simulink model "TST_CrCUI"  (R2016b)
settings: Solver=FixedStepDiscrete  StartTime=0.0  StopTime=simTime  FixedStep=sampleTime  RelTol=1e-3
values from neighbouring files (symbols this model uses):
  testCase = 1    [initTST_CrCUI_001.m]
libraries: simulink x4, UnitTest_Lib x1
settings Model: Creator=guanxiaoxing  LastModifiedBy=guanxiaoxing
settings DebuggingCC: SignalRangeChecking=error

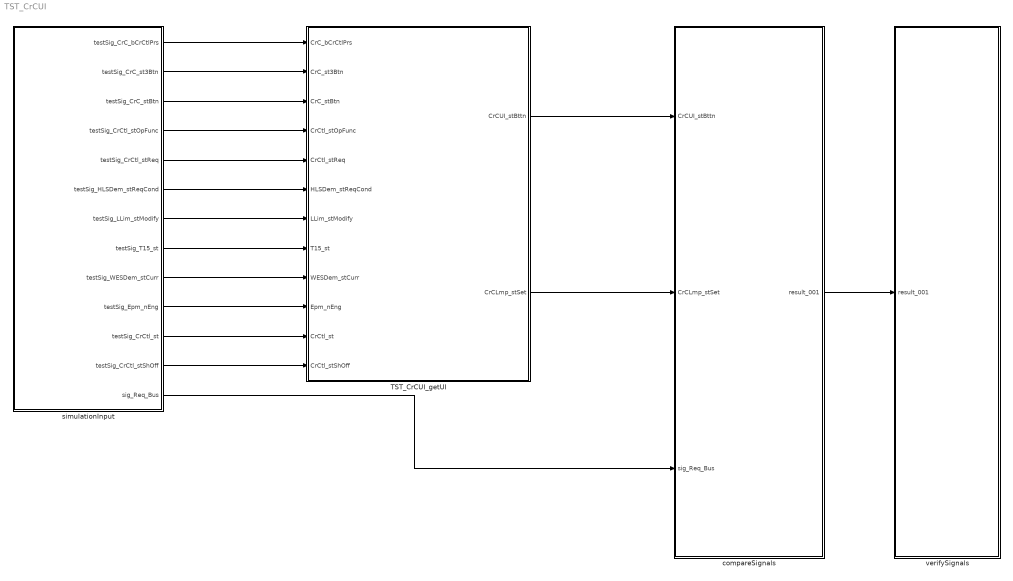
== system TST_CrCUI ==
  TST_CrCUI_getUI : Subsystem
  compareSignals : Subsystem
  simulationInput : Subsystem
  verifySignals : Subsystem
  wires:
  simulationInput/1(testSig_CrC_bCrCtlPrs) -> TST_CrCUI_getUI/1(CrC_bCrCtlPrs)
  simulationInput/2(testSig_CrC_st3Btn) -> TST_CrCUI_getUI/2(CrC_st3Btn)
  simulationInput/3(testSig_CrC_stBtn) -> TST_CrCUI_getUI/3(CrC_stBtn)
  simulationInput/4(testSig_CrCtl_stOpFunc) -> TST_CrCUI_getUI/4(CrCtl_stOpFunc)
  simulationInput/5(testSig_CrCtl_stReq) -> TST_CrCUI_getUI/5(CrCtl_stReq)
  simulationInput/6(testSig_HLSDem_stReqCond) -> TST_CrCUI_getUI/6(HLSDem_stReqCond)
  simulationInput/7(testSig_LLim_stModify) -> TST_CrCUI_getUI/7(LLim_stModify)
  simulationInput/8(testSig_T15_st) -> TST_CrCUI_getUI/8(T15_st)
  simulationInput/9(testSig_WESDem_stCurr) -> TST_CrCUI_getUI/9(WESDem_stCurr)
  simulationInput/10(testSig_Epm_nEng) -> TST_CrCUI_getUI/10(Epm_nEng)
  simulationInput/11(testSig_CrCtl_st) -> TST_CrCUI_getUI/11(CrCtl_st)
  simulationInput/12(testSig_CrCtl_stShOff) -> TST_CrCUI_getUI/12(CrCtl_stShOff)
  TST_CrCUI_getUI/1(CrCUI_stBttn) -> compareSignals/1(CrCUI_stBttn)
  TST_CrCUI_getUI/2(CrCLmp_stSet) -> compareSignals/2(CrCLmp_stSet)
  simulationInput/13(sig_Req_Bus) -> compareSignals/3(sig_Req_Bus)
  compareSignals/1(result_001) -> verifySignals/1(result_001)

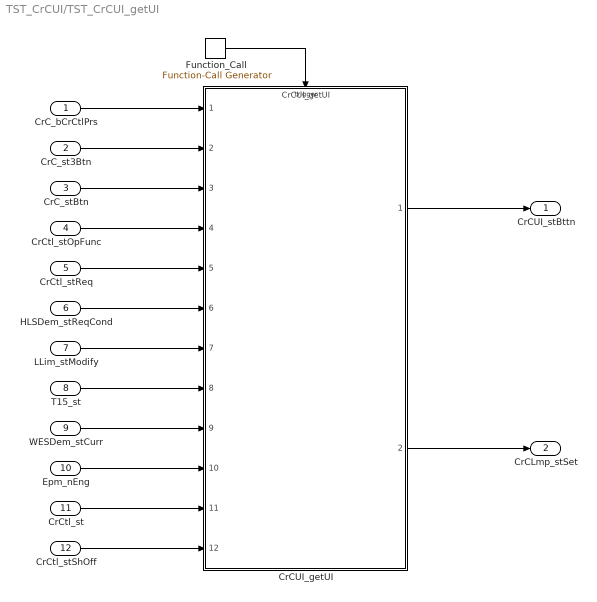
== system TST_CrCUI/TST_CrCUI_getUI ==
  CrC_bCrCtlPrs : Inport
  CrC_st3Btn : Inport  Port=2
  CrC_stBtn : Inport  Port=3
  CrCtl_stOpFunc : Inport  Port=4
  CrCtl_stReq : Inport  Port=5
  HLSDem_stReqCond : Inport  Port=6
  LLim_stModify : Inport  Port=7
  T15_st : Inport  Port=8
  WESDem_stCurr : Inport  Port=9
  Epm_nEng : Inport  Port=10
  CrCtl_st : Inport  Port=11
  CrCtl_stShOff : Inport  Port=12
  CrCUI_getUI : ModelReference  ModelNameDialog=CrCUI_getUI  SimulationMode=Normal  ModelReferenceVersion=1.56  TriggerPortName=function  TriggerPortTriggerType=function-call  TriggerPortStatesWhenEnabling=held
  Function_Call : simulink/Ports & Subsystems/Function-Call Generator  sample_time=sampleTime  numberOfIterations=1
  CrCUI_stBttn : Outport
  CrCLmp_stSet : Outport  Port=2
  wires:
  Function_Call/1 -> CrCUI_getUI/Trigger
  CrC_bCrCtlPrs/1 -> CrCUI_getUI/1
  CrC_st3Btn/1 -> CrCUI_getUI/2
  CrC_stBtn/1 -> CrCUI_getUI/3
  CrCtl_stOpFunc/1 -> CrCUI_getUI/4
  CrCtl_stReq/1 -> CrCUI_getUI/5
  HLSDem_stReqCond/1 -> CrCUI_getUI/6
  LLim_stModify/1 -> CrCUI_getUI/7
  T15_st/1 -> CrCUI_getUI/8
  WESDem_stCurr/1 -> CrCUI_getUI/9
  Epm_nEng/1 -> CrCUI_getUI/10
  CrCtl_st/1 -> CrCUI_getUI/11
  CrCtl_stShOff/1 -> CrCUI_getUI/12
  CrCUI_getUI/1 -> CrCUI_stBttn/1
  CrCUI_getUI/2 -> CrCLmp_stSet/1

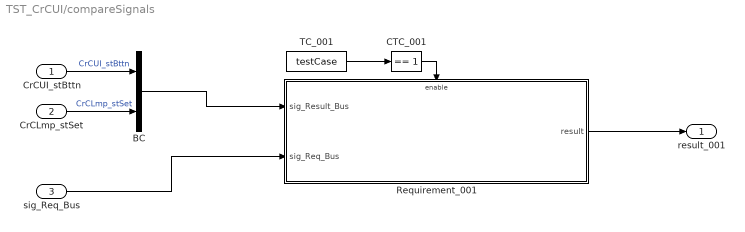
== system TST_CrCUI/compareSignals ==
  CrCUI_stBttn : Inport
  CrCLmp_stSet : Inport  Port=2
  sig_Req_Bus : Inport  Port=3
  BC : BusCreator  Inputs=2
  CTC_001 : simulink/Logic and Bit Operations/Compare To Constant  relop===  const=1  OutDataTypeStr=boolean
  Requirement_001 : Subsystem
  TC_001 : Constant  Value=testCase
  result_001 : Outport
  wires:
  CrCUI_stBttn/1 -> BC/1  "CrCUI_stBttn"
  CrCLmp_stSet/1 -> BC/2  "CrCLmp_stSet"
  TC_001/1 -> CTC_001/1
  CTC_001/1 -> Requirement_001/Enable
  sig_Req_Bus/1 -> Requirement_001/2(sig_Req_Bus)
  BC/1 -> Requirement_001/1(sig_Result_Bus)
  Requirement_001/1(result) -> result_001/1

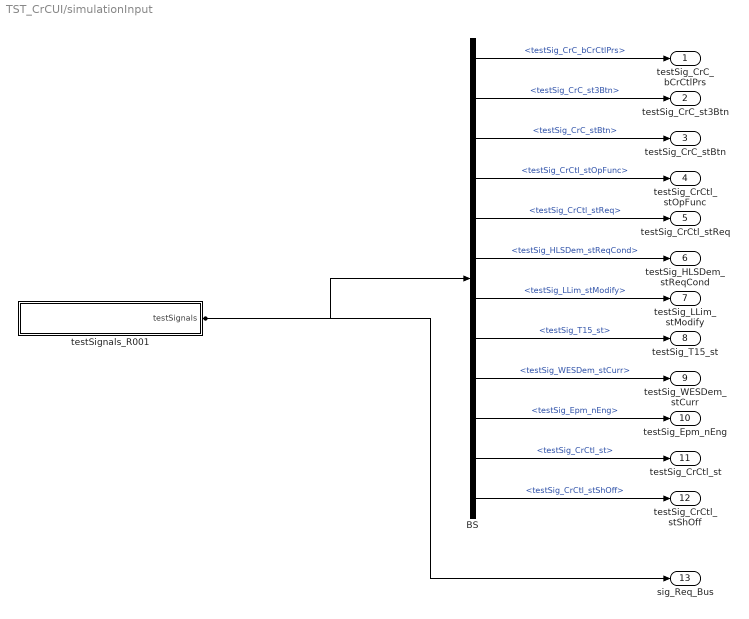
== system TST_CrCUI/simulationInput ==
  BS : BusSelector  OutputSignals=testSig_CrC_bCrCtlPrs,testSig_CrC_st3Btn,testSig_CrC_stBtn,testSig_CrCtl_stOpFunc,testSig_CrCtl_stReq,testSig_HLSDem_stReqCond,testSig_LLim_stModify,testSig_T15_st,testSig_WESDem_stCurr,testSig_Epm_nEng,testSig_CrCtl_st,testSig_CrCtl_stShOff
  testSignals_R001 : Subsystem
  testSig_CrC_bCrCtlPrs : Outport
  testSig_CrC_st3Btn : Outport  Port=2
  testSig_CrC_stBtn : Outport  Port=3
  testSig_CrCtl_stOpFunc : Outport  Port=4
  testSig_CrCtl_stReq : Outport  Port=5
  testSig_HLSDem_stReqCond : Outport  Port=6
  testSig_LLim_stModify : Outport  Port=7
  testSig_T15_st : Outport  Port=8
  testSig_WESDem_stCurr : Outport  Port=9
  testSig_Epm_nEng : Outport  Port=10
  testSig_CrCtl_st : Outport  Port=11
  testSig_CrCtl_stShOff : Outport  Port=12
  sig_Req_Bus : Outport  Port=13
  wires:
  BS/1 -> testSig_CrC_bCrCtlPrs/1  "<testSig_CrC_bCrCtlPrs>"
  BS/2 -> testSig_CrC_st3Btn/1  "<testSig_CrC_st3Btn>"
  BS/3 -> testSig_CrC_stBtn/1  "<testSig_CrC_stBtn>"
  BS/4 -> testSig_CrCtl_stOpFunc/1  "<testSig_CrCtl_stOpFunc>"
  BS/5 -> testSig_CrCtl_stReq/1  "<testSig_CrCtl_stReq>"
  BS/6 -> testSig_HLSDem_stReqCond/1  "<testSig_HLSDem_stReqCond>"
  BS/7 -> testSig_LLim_stModify/1  "<testSig_LLim_stModify>"
  BS/8 -> testSig_T15_st/1  "<testSig_T15_st>"
  BS/9 -> testSig_WESDem_stCurr/1  "<testSig_WESDem_stCurr>"
  BS/10 -> testSig_Epm_nEng/1  "<testSig_Epm_nEng>"
  BS/11 -> testSig_CrCtl_st/1  "<testSig_CrCtl_st>"
  BS/12 -> testSig_CrCtl_stShOff/1  "<testSig_CrCtl_stShOff>"
  testSignals_R001/1(testSignals) -> BS/1, sig_Req_Bus/1

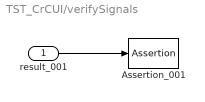
== system TST_CrCUI/verifySignals ==
  result_001 : Inport
  Assertion_001 : Assertion  Enabled=off
  wires:
  result_001/1 -> Assertion_001/1

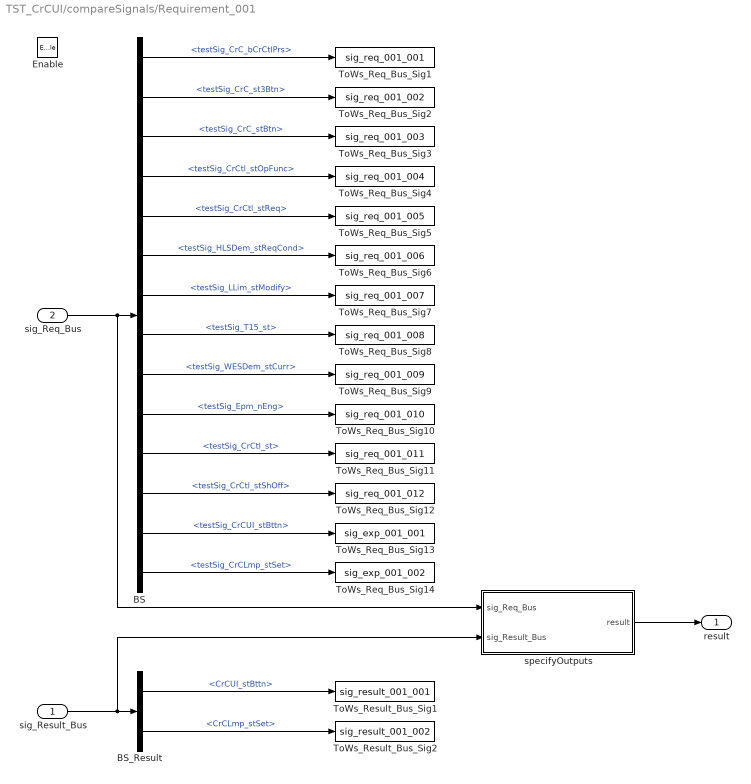
== system TST_CrCUI/compareSignals/Requirement_001 ==
  sig_Result_Bus : Inport
  sig_Req_Bus : Inport  Port=2
  Enable : EnablePort
  BS : BusSelector  OutputSignals=testSig_CrC_bCrCtlPrs,testSig_CrC_st3Btn,testSig_CrC_stBtn,testSig_CrCtl_stOpFunc,testSig_CrCtl_stReq,testSig_HLSDem_stReqCond,testSig_LLim_stModify,testSig_T15_st,testSig_WESDem_stCurr,testSig_Epm_nEng,testSig_CrCtl_st,testSig_CrCtl_stShOff,testSig_CrCUI_stBttn,testSig_CrCLmp_stSet
  BS_Result : BusSelector  OutputSignals=CrCUI_stBttn,CrCLmp_stSet
  ToWs_Req_Bus_Sig1 : ToWorkspace  VariableName=sig_req_001_001  SaveFormat=Structure With Time
  ToWs_Req_Bus_Sig10 : ToWorkspace  VariableName=sig_req_001_010  SaveFormat=Structure With Time
  ToWs_Req_Bus_Sig11 : ToWorkspace  VariableName=sig_req_001_011  SaveFormat=Structure With Time
  ToWs_Req_Bus_Sig12 : ToWorkspace  VariableName=sig_req_001_012  SaveFormat=Structure With Time
  ToWs_Req_Bus_Sig13 : ToWorkspace  VariableName=sig_exp_001_001  SaveFormat=Structure With Time
  ToWs_Req_Bus_Sig14 : ToWorkspace  VariableName=sig_exp_001_002  SaveFormat=Structure With Time
  ToWs_Req_Bus_Sig2 : ToWorkspace  VariableName=sig_req_001_002  SaveFormat=Structure With Time
  ToWs_Req_Bus_Sig3 : ToWorkspace  VariableName=sig_req_001_003  SaveFormat=Structure With Time
  ToWs_Req_Bus_Sig4 : ToWorkspace  VariableName=sig_req_001_004  SaveFormat=Structure With Time
  ToWs_Req_Bus_Sig5 : ToWorkspace  VariableName=sig_req_001_005  SaveFormat=Structure With Time
  ToWs_Req_Bus_Sig6 : ToWorkspace  VariableName=sig_req_001_006  SaveFormat=Structure With Time
  ToWs_Req_Bus_Sig7 : ToWorkspace  VariableName=sig_req_001_007  SaveFormat=Structure With Time
  ToWs_Req_Bus_Sig8 : ToWorkspace  VariableName=sig_req_001_008  SaveFormat=Structure With Time
  ToWs_Req_Bus_Sig9 : ToWorkspace  VariableName=sig_req_001_009  SaveFormat=Structure With Time
  ToWs_Result_Bus_Sig1 : ToWorkspace  VariableName=sig_result_001_001  SaveFormat=Structure With Time
  ToWs_Result_Bus_Sig2 : ToWorkspace  VariableName=sig_result_001_002  SaveFormat=Structure With Time
  specifyOutputs : Subsystem
  result : Outport
  wires:
  sig_Req_Bus/1 -> BS/1, specifyOutputs/1(sig_Req_Bus)
  BS/1 -> ToWs_Req_Bus_Sig1/1  "<testSig_CrC_bCrCtlPrs>"
  BS/2 -> ToWs_Req_Bus_Sig2/1  "<testSig_CrC_st3Btn>"
  BS/3 -> ToWs_Req_Bus_Sig3/1  "<testSig_CrC_stBtn>"
  BS/4 -> ToWs_Req_Bus_Sig4/1  "<testSig_CrCtl_stOpFunc>"
  BS/5 -> ToWs_Req_Bus_Sig5/1  "<testSig_CrCtl_stReq>"
  BS/6 -> ToWs_Req_Bus_Sig6/1  "<testSig_HLSDem_stReqCond>"
  BS/7 -> ToWs_Req_Bus_Sig7/1  "<testSig_LLim_stModify>"
  BS/8 -> ToWs_Req_Bus_Sig8/1  "<testSig_T15_st>"
  BS/9 -> ToWs_Req_Bus_Sig9/1  "<testSig_WESDem_stCurr>"
  BS/10 -> ToWs_Req_Bus_Sig10/1  "<testSig_Epm_nEng>"
  BS/11 -> ToWs_Req_Bus_Sig11/1  "<testSig_CrCtl_st>"
  BS/12 -> ToWs_Req_Bus_Sig12/1  "<testSig_CrCtl_stShOff>"
  BS/13 -> ToWs_Req_Bus_Sig13/1  "<testSig_CrCUI_stBttn>"
  BS/14 -> ToWs_Req_Bus_Sig14/1  "<testSig_CrCLmp_stSet>"
  sig_Result_Bus/1 -> BS_Result/1, specifyOutputs/2(sig_Result_Bus)
  BS_Result/1 -> ToWs_Result_Bus_Sig1/1  "<CrCUI_stBttn>"
  BS_Result/2 -> ToWs_Result_Bus_Sig2/1  "<CrCLmp_stSet>"
  specifyOutputs/1(result) -> result/1

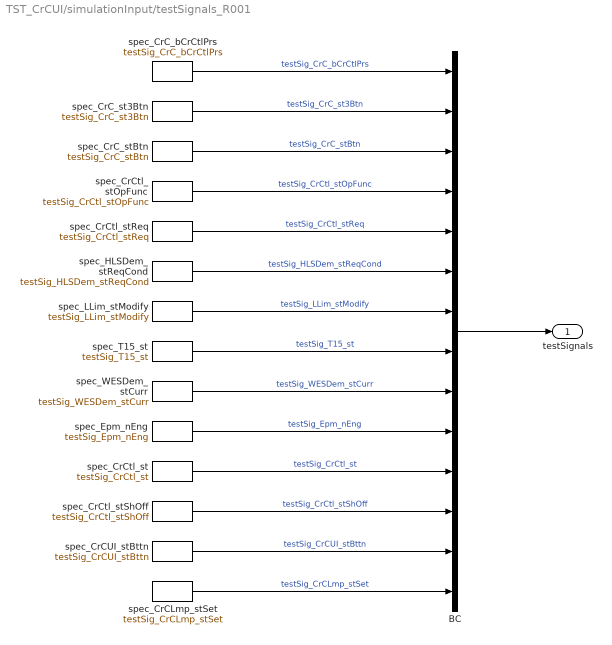
== system TST_CrCUI/simulationInput/testSignals_R001 ==
  BC : BusCreator  Inputs=14
  spec_CrCLmp_stSet : FromWorkspace  VariableName=testSig_CrCLmp_stSet  Interpolate=off  OutputAfterFinalValue=Holding final value
  spec_CrCUI_stBttn : FromWorkspace  VariableName=testSig_CrCUI_stBttn  Interpolate=off  OutputAfterFinalValue=Holding final value
  spec_CrC_bCrCtlPrs : FromWorkspace  VariableName=testSig_CrC_bCrCtlPrs  Interpolate=off  OutputAfterFinalValue=Holding final value
  spec_CrC_st3Btn : FromWorkspace  VariableName=testSig_CrC_st3Btn  Interpolate=off  OutputAfterFinalValue=Holding final value
  spec_CrC_stBtn : FromWorkspace  VariableName=testSig_CrC_stBtn  Interpolate=off  OutputAfterFinalValue=Holding final value
  spec_CrCtl_st : FromWorkspace  VariableName=testSig_CrCtl_st  Interpolate=off  OutputAfterFinalValue=Holding final value
  spec_CrCtl_stOpFunc : FromWorkspace  VariableName=testSig_CrCtl_stOpFunc  Interpolate=off  OutputAfterFinalValue=Holding final value
  spec_CrCtl_stReq : FromWorkspace  VariableName=testSig_CrCtl_stReq  Interpolate=off  OutputAfterFinalValue=Holding final value
  spec_CrCtl_stShOff : FromWorkspace  VariableName=testSig_CrCtl_stShOff  Interpolate=off  OutputAfterFinalValue=Holding final value
  spec_Epm_nEng : FromWorkspace  VariableName=testSig_Epm_nEng  Interpolate=off  OutputAfterFinalValue=Holding final value
  spec_HLSDem_stReqCond : FromWorkspace  VariableName=testSig_HLSDem_stReqCond  Interpolate=off  OutputAfterFinalValue=Holding final value
  spec_LLim_stModify : FromWorkspace  VariableName=testSig_LLim_stModify  Interpolate=off  OutputAfterFinalValue=Holding final value
  spec_T15_st : FromWorkspace  VariableName=testSig_T15_st  Interpolate=off  OutputAfterFinalValue=Holding final value
  spec_WESDem_stCurr : FromWorkspace  VariableName=testSig_WESDem_stCurr  Interpolate=off  OutputAfterFinalValue=Holding final value
  testSignals : Outport
  wires:
  BC/1 -> testSignals/1
  spec_CrC_bCrCtlPrs/1 -> BC/1  "testSig_CrC_bCrCtlPrs"
  spec_CrC_st3Btn/1 -> BC/2  "testSig_CrC_st3Btn"
  spec_CrC_stBtn/1 -> BC/3  "testSig_CrC_stBtn"
  spec_CrCtl_stOpFunc/1 -> BC/4  "testSig_CrCtl_stOpFunc"
  spec_CrCtl_stReq/1 -> BC/5  "testSig_CrCtl_stReq"
  spec_HLSDem_stReqCond/1 -> BC/6  "testSig_HLSDem_stReqCond"
  spec_LLim_stModify/1 -> BC/7  "testSig_LLim_stModify"
  spec_T15_st/1 -> BC/8  "testSig_T15_st"
  spec_WESDem_stCurr/1 -> BC/9  "testSig_WESDem_stCurr"
  spec_Epm_nEng/1 -> BC/10  "testSig_Epm_nEng"
  spec_CrCtl_st/1 -> BC/11  "testSig_CrCtl_st"
  spec_CrCtl_stShOff/1 -> BC/12  "testSig_CrCtl_stShOff"
  spec_CrCUI_stBttn/1 -> BC/13  "testSig_CrCUI_stBttn"
  spec_CrCLmp_stSet/1 -> BC/14  "testSig_CrCLmp_stSet"

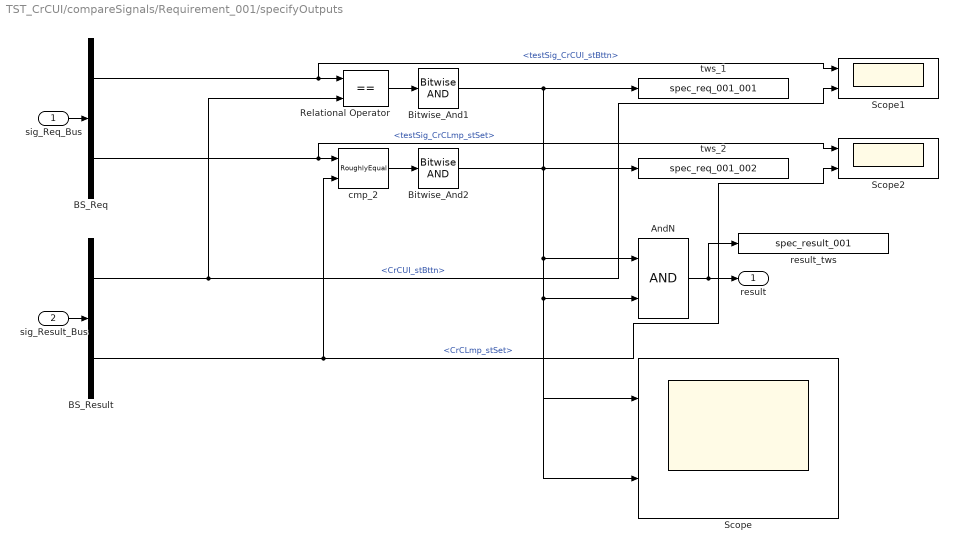
== system TST_CrCUI/compareSignals/Requirement_001/specifyOutputs ==
  sig_Req_Bus : Inport
  sig_Result_Bus : Inport  Port=2
  AndN : Logic
  BS_Req : BusSelector  OutputSignals=testSig_CrCUI_stBttn,testSig_CrCLmp_stSet
  BS_Result : BusSelector  OutputSignals=CrCUI_stBttn,CrCLmp_stSet
  Bitwise_And1 : simulink/Logic and Bit Operations/Bitwise Operator  logicop=AND  UseBitMask=off  BitMask=bin2dec('11011001')  BitMaskRealWorld=Stored Integer
  Bitwise_And2 : simulink/Logic and Bit Operations/Bitwise Operator  logicop=AND  UseBitMask=off  BitMask=bin2dec('11011001')  BitMaskRealWorld=Stored Integer
  Relational Operator : RelationalOperator  Operator===  OutDataTypeStr=boolean  RndMeth=Simplest
  Scope : Scope  NumInputPorts=2
  Scope1 : Scope  NumInputPorts=2
  Scope2 : Scope  NumInputPorts=2
  cmp_2 : UnitTest_Lib/RoughlyEqual  slope=0.1
  result_tws : ToWorkspace  VariableName=spec_result_001
  tws_1 : ToWorkspace  VariableName=spec_req_001_001
  tws_2 : ToWorkspace  VariableName=spec_req_001_002
  result : Outport
  wires:
  sig_Req_Bus/1 -> BS_Req/1
  sig_Result_Bus/1 -> BS_Result/1
  AndN/1 -> result/1, result_tws/1
  BS_Req/1 -> Relational Operator/1, Scope1/1  "<testSig_CrCUI_stBttn>"
  BS_Result/1 -> Relational Operator/2, Scope1/2  "<CrCUI_stBttn>"
  Relational Operator/1 -> Bitwise_And1/1
  Bitwise_And1/1 -> AndN/1, Scope/1, tws_1/1
  BS_Req/2 -> cmp_2/1, Scope2/1  "<testSig_CrCLmp_stSet>"
  BS_Result/2 -> cmp_2/2, Scope2/2  "<CrCLmp_stSet>"
  cmp_2/1 -> Bitwise_And2/1
  Bitwise_And2/1 -> AndN/2, Scope/2, tws_2/1
